simulink model "brakeSystemNeuralNetworkSimulink19b"  (R2021b)
settings: Solver=VariableStepAuto  StartTime=0.0  StopTime=25.0  RelTol=1e-3
settings Model: Creator=hgrady  LastModifiedBy=Nick
settings SolverCC: AlgebraicLoopSolver=TrustRegion

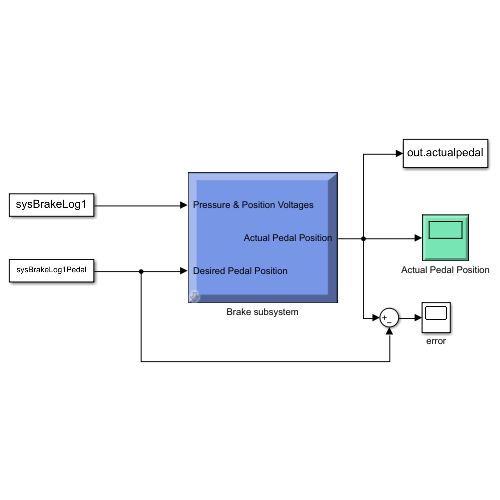
[thumbnail: Simulink's stored preview of the top-level diagram]
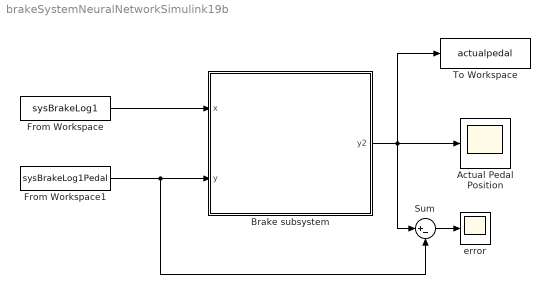
== system brakeSystemNeuralNetworkSimulink19b ==
  Actual Pedal Position : Scope
      mask Display: e = 0.06;c1 = [120 230 180]/255;c2 = ([120 230 180]+0)/(256+128);c3 = ([120 230 180]+128)/(256+128);patch([0 1 1 0],[0 0 1 1],c1);patch([0 1 1 1-e 1-e 0+e],[0 0 1 1-e 0+e 0+e],c2);patch([0 0 1 1-e 0+e 0+e],[0 1 1 1-e 1-e 0+e],c3);plot([0 1 1 0 0],[0 0 1 1 0]);plot([0.15 0.85 0.85 0.15 0.15],[0.5 0.5 0.85 0.85 0.5]);
  Brake subsystem : Subsystem  mask{pi_input_1_delayed_1=[0;0;0;0], pi_input_1_delayed_2=[0;0;0;0], pi_input_1_delayed_3=[0;0;0;0], pi_input_1_delayed_4=[0;0;0;0], pi_input_2_delayed_1=0, pi_input_2_delayed_2=0, pi_input_2_delayed_3=0, pi_input_2_delayed_4=0}
      mask prompts: pi_input_1_delayed_1 "Preprocessed initial input 1 state at timestep 0."; pi_input_1_delayed_2 "Preprocessed initial input 1 state at timestep -1."; pi_input_1_delayed_3 "Preprocessed initial input 1 state at timestep -2."; pi_input_1_delayed_4 "Preprocessed initial input 1 state at timestep -3."; pi_input_2_delayed_1 "Preprocessed initial input 2 state at timestep 0."; pi_input_2_delayed_2 "Preprocessed initial input 2 state at timestep -1."; pi_input_2_delayed_3 "Preprocessed initial input 2 state at timestep -2."; pi_input_2_delayed_4 "Preprocessed initial input 2 state at timestep -3."
      mask help: NARX Neural Network
      mask Display: e = 0.06;c1 = [120 150 230]/255;c2 = ([120 150 230]+0)/383;c3 = ([120 150 230]+128)/383;patch([0 1 1 0],[0 0 1 1],c1);patch([0 1 1 1-e 1-e 0+e],[0 0 1 1-e 0+e 0+e],c2);patch([0 0 1 1-e 0+e 0+e],[0 1 1 1-e 1-e 0+e],c3);plot([0 1 1 0 0],[0 0 1 1 0]);fprintf('');port_label('input',1,' Pressure & Position Voltages');port_label('input',2,' Desired Pedal Position');port_label('output',1,'Actual Pedal Position ');
  From Workspace : FromWorkspace  VariableName=sysBrakeLog1  SampleTime=0.033
  From Workspace1 : FromWorkspace  VariableName=sysBrakeLog1Pedal  SampleTime=0.033
  Sum : Sum  Inputs=|+-
  To Workspace : ToWorkspace  VariableName=actualpedal  SaveFormat=Timeseries  SampleTime=-1
  error : Scope
  wires:
  Brake subsystem/1(y2) -> To Workspace/1, Actual Pedal Position/1, Sum/1
  Sum/1 -> error/1
  From Workspace/1 -> Brake subsystem/1(x)
  From Workspace1/1 -> Brake subsystem/2(y), Sum/2

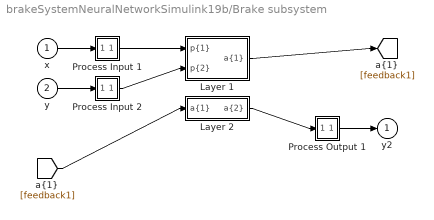
== system brakeSystemNeuralNetworkSimulink19b/Brake subsystem ==
  x : Inport  PortDimensions=4
      mask Display: e = 0.06;c1 = [120 230 180]/255;c2 = ([120 230 180]+0)/(256+128);c3 = ([120 230 180]+128)/(256+128);patch([0 1 1 0],[0 0 1 1],c1);patch([0 1 1 1-e 1-e 0+e],[0 0 1 1-e 0+e 0+e],c2);patch([0 0 1 1-e 0+e 0+e],[0 1 1 1-e 1-e 0+e],c3);plot([0 1 1 0 0],[0 0 1 1 0]);
  y : Inport  Port=2  PortDimensions=1
      mask Display: e = 0.06;c1 = [120 230 180]/255;c2 = ([120 230 180]+0)/(256+128);c3 = ([120 230 180]+128)/(256+128);patch([0 1 1 0],[0 0 1 1],c1);patch([0 1 1 1-e 1-e 0+e],[0 0 1 1-e 0+e 0+e],c2);patch([0 0 1 1-e 0+e 0+e],[0 1 1 1-e 1-e 0+e],c3);plot([0 1 1 0 0],[0 0 1 1 0]);
  Layer 1 : Subsystem
      mask Display: e = 0.06;c1 = [120 150 230]/255;c2 = ([120 150 230]+0)/383;c3 = ([120 150 230]+128)/383;patch([0 1 1 0],[0 0 1 1],c1);patch([0 1 1 1-e 1-e 0+e],[0 0 1 1-e 0+e 0+e],c2);patch([0 0 1 1-e 0+e 0+e],[0 1 1 1-e 1-e 0+e],c3);plot([0 1 1 0 0],[0 0 1 1 0]);
  Layer 2 : Subsystem
      mask Display: e = 0.06;c1 = [120 150 230]/255;c2 = ([120 150 230]+0)/383;c3 = ([120 150 230]+128)/383;patch([0 1 1 0],[0 0 1 1],c1);patch([0 1 1 1-e 1-e 0+e],[0 0 1 1-e 0+e 0+e],c2);patch([0 0 1 1-e 0+e 0+e],[0 1 1 1-e 1-e 0+e],c3);plot([0 1 1 0 0],[0 0 1 1 0]);
  Process Input 1 : Subsystem
      mask Display: e = 0.06;c1 = [120 150 230]/255;c2 = ([120 150 230]+0)/383;c3 = ([120 150 230]+128)/383;patch([0 1 1 0],[0 0 1 1],c1);patch([0 1 1 1-e 1-e 0+e],[0 0 1 1-e 0+e 0+e],c2);patch([0 0 1 1-e 0+e 0+e],[0 1 1 1-e 1-e 0+e],c3);plot([0 1 1 0 0],[0 0 1 1 0]);
  Process Input 2 : Subsystem
      mask Display: e = 0.06;c1 = [120 150 230]/255;c2 = ([120 150 230]+0)/383;c3 = ([120 150 230]+128)/383;patch([0 1 1 0],[0 0 1 1],c1);patch([0 1 1 1-e 1-e 0+e],[0 0 1 1-e 0+e 0+e],c2);patch([0 0 1 1-e 0+e 0+e],[0 1 1 1-e 1-e 0+e],c3);plot([0 1 1 0 0],[0 0 1 1 0]);
  Process Output 1 : Subsystem
      mask Display: e = 0.06;c1 = [120 150 230]/255;c2 = ([120 150 230]+0)/383;c3 = ([120 150 230]+128)/383;patch([0 1 1 0],[0 0 1 1],c1);patch([0 1 1 1-e 1-e 0+e],[0 0 1 1-e 0+e 0+e],c2);patch([0 0 1 1-e 0+e 0+e],[0 1 1 1-e 1-e 0+e],c3);plot([0 1 1 0 0],[0 0 1 1 0]);
  y2 : Outport  InitialOutput=0
      mask Display: e = 0.06;c1 = [120 230 180]/255;c2 = ([120 230 180]+0)/(256+128);c3 = ([120 230 180]+128)/(256+128);patch([0 1 1 0],[0 0 1 1],c1);patch([0 1 1 1-e 1-e 0+e],[0 0 1 1-e 0+e 0+e],c2);patch([0 0 1 1-e 0+e 0+e],[0 1 1 1-e 1-e 0+e],c3);plot([0 1 1 0 0],[0 0 1 1 0]);
  wires:
  x/1 -> Process Input 1/1(x)
  y/1 -> Process Input 2/1(x)
  Process Output 1/1(y) -> y2/1
  Process Input 1/1(p) -> Layer 1/1("p{1}")
  Process Input 2/1(p) -> Layer 1/2("p{2}")
  Layer 1/1("a{1}") -> [feedback1]
  [feedback1] -> Layer 2/1("a{1} ")
  Layer 2/1("a{2}") -> Process Output 1/1(a)

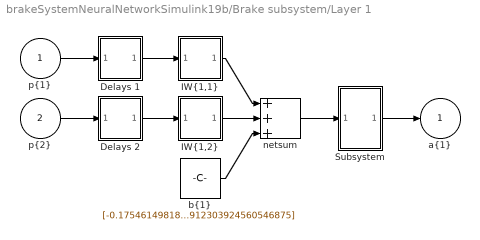
== system brakeSystemNeuralNetworkSimulink19b/Brake subsystem/Layer 1 ==
  "p{1}" : Inport  PortDimensions=4
      mask Display: e = 0.06;c1 = [120 230 180]/255;c2 = ([120 230 180]+0)/(256+128);c3 = ([120 230 180]+128)/(256+128);patch([0 1 1 0],[0 0 1 1],c1);patch([0 1 1 1-e 1-e 0+e],[0 0 1 1-e 0+e 0+e],c2);patch([0 0 1 1-e 0+e 0+e],[0 1 1 1-e 1-e 0+e],c3);plot([0 1 1 0 0],[0 0 1 1 0]);
  "p{2}" : Inport  Port=2  PortDimensions=1
      mask Display: e = 0.06;c1 = [120 230 180]/255;c2 = ([120 230 180]+0)/(256+128);c3 = ([120 230 180]+128)/(256+128);patch([0 1 1 0],[0 0 1 1],c1);patch([0 1 1 1-e 1-e 0+e],[0 0 1 1-e 0+e 0+e],c2);patch([0 0 1 1-e 0+e 0+e],[0 1 1 1-e 1-e 0+e],c3);plot([0 1 1 0 0],[0 0 1 1 0]);
  Delays 1 : Subsystem
      mask Display: e = 0.06;c1 = [120 150 230]/255;c2 = ([120 150 230]+0)/383;c3 = ([120 150 230]+128)/383;patch([0 1 1 0],[0 0 1 1],c1);patch([0 1 1 1-e 1-e 0+e],[0 0 1 1-e 0+e 0+e],c2);patch([0 0 1 1-e 0+e 0+e],[0 1 1 1-e 1-e 0+e],c3);plot([0 1 1 0 0],[0 0 1 1 0]);disp('1-4');
  Delays 2 : Subsystem
      mask Display: e = 0.06;c1 = [120 150 230]/255;c2 = ([120 150 230]+0)/383;c3 = ([120 150 230]+128)/383;patch([0 1 1 0],[0 0 1 1],c1);patch([0 1 1 1-e 1-e 0+e],[0 0 1 1-e 0+e 0+e],c2);patch([0 0 1 1-e 0+e 0+e],[0 1 1 1-e 1-e 0+e],c3);plot([0 1 1 0 0],[0 0 1 1 0]);disp('1-4');
  "IW{1,1}" : Subsystem
      mask Display: e = 0.06;c1 = [120 150 230]/255;c2 = ([120 150 230]+0)/383;c3 = ([120 150 230]+128)/383;patch([0 1 1 0],[0 0 1 1],c1);patch([0 1 1 1-e 1-e 0+e],[0 0 1 1-e 0+e 0+e],c2);patch([0 0 1 1-e 0+e 0+e],[0 1 1 1-e 1-e 0+e],c3);plot([0 1 1 0 0],[0 0 1 1 0]);disp('W');
  "IW{1,2}" : Subsystem
      mask Display: e = 0.06;c1 = [120 150 230]/255;c2 = ([120 150 230]+0)/383;c3 = ([120 150 230]+128)/383;patch([0 1 1 0],[0 0 1 1],c1);patch([0 1 1 1-e 1-e 0+e],[0 0 1 1-e 0+e 0+e],c2);patch([0 0 1 1-e 0+e 0+e],[0 1 1 1-e 1-e 0+e],c3);plot([0 1 1 0 0],[0 0 1 1 0]);disp('W');
  Subsystem : Subsystem
  "b{1}" : Constant  Value=[-0.1754614981831461861805365742839057929813861846923828125;0.1568951812336805973213671450139372609555721282958984375;0.092589380084686812022454205362009815871715545654296875;-0.08827103518596403353146939707585261203348636627197265625;-0.1366947078190251796403487105635576881468296051025390625;-1.6956623977816700499232638321700505912303924560546875]
      mask Display: e = 0.06;c1 = [120 150 230]/255;c2 = ([120 150 230]+0)/383;c3 = ([120 150 230]+128)/383;patch([0 1 1 0],[0 0 1 1],c1);patch([0 1 1 1-e 1-e 0+e],[0 0 1 1-e 0+e 0+e],c2);patch([0 0 1 1-e 0+e 0+e],[0 1 1 1-e 1-e 0+e],c3);plot([0 1 1 0 0],[0 0 1 1 0]);disp('b');
  netsum : Sum  Inputs=3  InputSameDT=on  SaturateOnIntegerOverflow=on  OutDataTypeStr=Inherit: Same as first input
      mask Display: e = 0.06;c1 = [120 150 230]/255;c2 = ([120 150 230]+0)/383;c3 = ([120 150 230]+128)/383;patch([0 1 1 0],[0 0 1 1],c1);patch([0 1 1 1-e 1-e 0+e],[0 0 1 1-e 0+e 0+e],c2);patch([0 0 1 1-e 0+e 0+e],[0 1 1 1-e 1-e 0+e],c3);plot([0 1 1 0 0],[0 0 1 1 0]);disp('+');
  "a{1}" : Outport  InitialOutput=[0;0;0;0;0;0]
      mask Display: e = 0.06;c1 = [120 230 180]/255;c2 = ([120 230 180]+0)/(256+128);c3 = ([120 230 180]+128)/(256+128);patch([0 1 1 0],[0 0 1 1],c1);patch([0 1 1 1-e 1-e 0+e],[0 0 1 1-e 0+e 0+e],c2);patch([0 0 1 1-e 0+e 0+e],[0 1 1 1-e 1-e 0+e],c3);plot([0 1 1 0 0],[0 0 1 1 0]);
  wires:
  "p{1}"/1 -> Delays 1/1("p{1}")
  Delays 1/1("pd{1,1}") -> "IW{1,1}"/1("pd{1,1}")
  "IW{1,1}"/1("iz{1,1}") -> netsum/1
  "p{2}"/1 -> Delays 2/1("p{1}")
  Delays 2/1("pd{1,2}") -> "IW{1,2}"/1("pd{1,2}")
  "IW{1,2}"/1("iz{1,2}") -> netsum/2
  "b{1}"/1 -> netsum/3
  netsum/1 -> Subsystem/1(In1)
  Subsystem/1("a{1}") -> "a{1}"/1

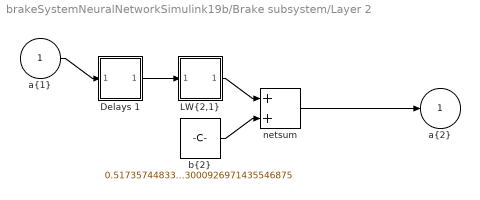
== system brakeSystemNeuralNetworkSimulink19b/Brake subsystem/Layer 2 ==
  "a{1} " : Inport  PortDimensions=6
      mask Display: e = 0.06;c1 = [120 230 180]/255;c2 = ([120 230 180]+0)/(256+128);c3 = ([120 230 180]+128)/(256+128);patch([0 1 1 0],[0 0 1 1],c1);patch([0 1 1 1-e 1-e 0+e],[0 0 1 1-e 0+e 0+e],c2);patch([0 0 1 1-e 0+e 0+e],[0 1 1 1-e 1-e 0+e],c3);plot([0 1 1 0 0],[0 0 1 1 0]);
  Delays 1 : Subsystem
      mask Display: e = 0.06;c1 = [120 150 230]/255;c2 = ([120 150 230]+0)/383;c3 = ([120 150 230]+128)/383;patch([0 1 1 0],[0 0 1 1],c1);patch([0 1 1 1-e 1-e 0+e],[0 0 1 1-e 0+e 0+e],c2);patch([0 0 1 1-e 0+e 0+e],[0 1 1 1-e 1-e 0+e],c3);plot([0 1 1 0 0],[0 0 1 1 0]);disp('0');
  "LW{2,1}" : Subsystem
      mask Display: e = 0.06;c1 = [120 150 230]/255;c2 = ([120 150 230]+0)/383;c3 = ([120 150 230]+128)/383;patch([0 1 1 0],[0 0 1 1],c1);patch([0 1 1 1-e 1-e 0+e],[0 0 1 1-e 0+e 0+e],c2);patch([0 0 1 1-e 0+e 0+e],[0 1 1 1-e 1-e 0+e],c3);plot([0 1 1 0 0],[0 0 1 1 0]);disp('W');
  "b{2}" : Constant  Value=0.51735744833768204653523525848868303000926971435546875
      mask Display: e = 0.06;c1 = [120 150 230]/255;c2 = ([120 150 230]+0)/383;c3 = ([120 150 230]+128)/383;patch([0 1 1 0],[0 0 1 1],c1);patch([0 1 1 1-e 1-e 0+e],[0 0 1 1-e 0+e 0+e],c2);patch([0 0 1 1-e 0+e 0+e],[0 1 1 1-e 1-e 0+e],c3);plot([0 1 1 0 0],[0 0 1 1 0]);disp('b');
  netsum : Sum  Inputs=2  InputSameDT=on  SaturateOnIntegerOverflow=on  OutDataTypeStr=Inherit: Same as first input
      mask Display: e = 0.06;c1 = [120 150 230]/255;c2 = ([120 150 230]+0)/383;c3 = ([120 150 230]+128)/383;patch([0 1 1 0],[0 0 1 1],c1);patch([0 1 1 1-e 1-e 0+e],[0 0 1 1-e 0+e 0+e],c2);patch([0 0 1 1-e 0+e 0+e],[0 1 1 1-e 1-e 0+e],c3);plot([0 1 1 0 0],[0 0 1 1 0]);disp('+');
  "a{2}" : Outport  InitialOutput=0
      mask Display: e = 0.06;c1 = [120 230 180]/255;c2 = ([120 230 180]+0)/(256+128);c3 = ([120 230 180]+128)/(256+128);patch([0 1 1 0],[0 0 1 1],c1);patch([0 1 1 1-e 1-e 0+e],[0 0 1 1-e 0+e 0+e],c2);patch([0 0 1 1-e 0+e 0+e],[0 1 1 1-e 1-e 0+e],c3);plot([0 1 1 0 0],[0 0 1 1 0]);
  wires:
  "a{1} "/1 -> Delays 1/1("p{2}")
  Delays 1/1("pd{2,1}") -> "LW{2,1}"/1("ad{2,1}")
  "LW{2,1}"/1("lz{2,1}") -> netsum/1
  "b{2}"/1 -> netsum/2
  netsum/1 -> "a{2}"/1

== system brakeSystemNeuralNetworkSimulink19b/Brake subsystem/Process Input 1 ==
  x : Inport  PortDimensions=4
      mask Display: e = 0.06;c1 = [120 230 180]/255;c2 = ([120 230 180]+0)/(256+128);c3 = ([120 230 180]+128)/(256+128);patch([0 1 1 0],[0 0 1 1],c1);patch([0 1 1 1-e 1-e 0+e],[0 0 1 1-e 0+e 0+e],c2);patch([0 0 1 1-e 0+e 0+e],[0 1 1 1-e 1-e 0+e],c3);plot([0 1 1 0 0],[0 0 1 1 0]);
  Subsystem : Subsystem
  p : Outport  PortDimensions=4
      mask Display: e = 0.06;c1 = [120 230 180]/255;c2 = ([120 230 180]+0)/(256+128);c3 = ([120 230 180]+128)/(256+128);patch([0 1 1 0],[0 0 1 1],c1);patch([0 1 1 1-e 1-e 0+e],[0 0 1 1-e 0+e 0+e],c2);patch([0 0 1 1-e 0+e 0+e],[0 1 1 1-e 1-e 0+e],c3);plot([0 1 1 0 0],[0 0 1 1 0]);
  wires:
  x/1 -> Subsystem/1(x)
  Subsystem/1(p) -> p/1

== system brakeSystemNeuralNetworkSimulink19b/Brake subsystem/Process Input 2 ==
  x : Inport  PortDimensions=1
      mask Display: e = 0.06;c1 = [120 230 180]/255;c2 = ([120 230 180]+0)/(256+128);c3 = ([120 230 180]+128)/(256+128);patch([0 1 1 0],[0 0 1 1],c1);patch([0 1 1 1-e 1-e 0+e],[0 0 1 1-e 0+e 0+e],c2);patch([0 0 1 1-e 0+e 0+e],[0 1 1 1-e 1-e 0+e],c3);plot([0 1 1 0 0],[0 0 1 1 0]);
  Subsystem : Subsystem
  p : Outport  PortDimensions=1
      mask Display: e = 0.06;c1 = [120 230 180]/255;c2 = ([120 230 180]+0)/(256+128);c3 = ([120 230 180]+128)/(256+128);patch([0 1 1 0],[0 0 1 1],c1);patch([0 1 1 1-e 1-e 0+e],[0 0 1 1-e 0+e 0+e],c2);patch([0 0 1 1-e 0+e 0+e],[0 1 1 1-e 1-e 0+e],c3);plot([0 1 1 0 0],[0 0 1 1 0]);
  wires:
  Subsystem/1(p) -> p/1
  x/1 -> Subsystem/1(x)

== system brakeSystemNeuralNetworkSimulink19b/Brake subsystem/Process Output 1 ==
  a : Inport  PortDimensions=1
      mask Display: e = 0.06;c1 = [120 230 180]/255;c2 = ([120 230 180]+0)/(256+128);c3 = ([120 230 180]+128)/(256+128);patch([0 1 1 0],[0 0 1 1],c1);patch([0 1 1 1-e 1-e 0+e],[0 0 1 1-e 0+e 0+e],c2);patch([0 0 1 1-e 0+e 0+e],[0 1 1 1-e 1-e 0+e],c3);plot([0 1 1 0 0],[0 0 1 1 0]);
  Subsystem : Subsystem
  y : Outport  PortDimensions=1
      mask Display: e = 0.06;c1 = [120 230 180]/255;c2 = ([120 230 180]+0)/(256+128);c3 = ([120 230 180]+128)/(256+128);patch([0 1 1 0],[0 0 1 1],c1);patch([0 1 1 1-e 1-e 0+e],[0 0 1 1-e 0+e 0+e],c2);patch([0 0 1 1-e 0+e 0+e],[0 1 1 1-e 1-e 0+e],c3);plot([0 1 1 0 0],[0 0 1 1 0]);
  wires:
  a/1 -> Subsystem/1(a)
  Subsystem/1(y) -> y/1

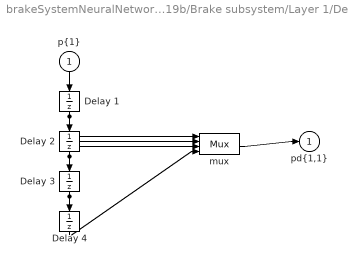
== system brakeSystemNeuralNetworkSimulink19b/Brake subsystem/Layer 1/Delays 1 ==
  "p{1}" : Inport  PortDimensions=4
      mask Display: e = 0.06;c1 = [120 230 180]/255;c2 = ([120 230 180]+0)/(256+128);c3 = ([120 230 180]+128)/(256+128);patch([0 1 1 0],[0 0 1 1],c1);patch([0 1 1 1-e 1-e 0+e],[0 0 1 1-e 0+e 0+e],c2);patch([0 0 1 1-e 0+e 0+e],[0 1 1 1-e 1-e 0+e],c3);plot([0 1 1 0 0],[0 0 1 1 0]);
  Delay 1 : UnitDelay  InitialCondition=pi_input_1_delayed_1  SampleTime=-1
      mask Display: e = 0.06;c1 = [120 150 230]/255;c2 = ([120 150 230]+0)/383;c3 = ([120 150 230]+128)/383;patch([0 1 1 0],[0 0 1 1],c1);patch([0 1 1 1-e 1-e 0+e],[0 0 1 1-e 0+e 0+e],c2);patch([0 0 1 1-e 0+e 0+e],[0 1 1 1-e 1-e 0+e],c3);plot([0 1 1 0 0],[0 0 1 1 0]);disp('D')
  Delay 2 : UnitDelay  InitialCondition=pi_input_1_delayed_2  SampleTime=-1
      mask Display: e = 0.06;c1 = [120 150 230]/255;c2 = ([120 150 230]+0)/383;c3 = ([120 150 230]+128)/383;patch([0 1 1 0],[0 0 1 1],c1);patch([0 1 1 1-e 1-e 0+e],[0 0 1 1-e 0+e 0+e],c2);patch([0 0 1 1-e 0+e 0+e],[0 1 1 1-e 1-e 0+e],c3);plot([0 1 1 0 0],[0 0 1 1 0]);disp('D')
  Delay 3 : UnitDelay  InitialCondition=pi_input_1_delayed_3  SampleTime=-1
      mask Display: e = 0.06;c1 = [120 150 230]/255;c2 = ([120 150 230]+0)/383;c3 = ([120 150 230]+128)/383;patch([0 1 1 0],[0 0 1 1],c1);patch([0 1 1 1-e 1-e 0+e],[0 0 1 1-e 0+e 0+e],c2);patch([0 0 1 1-e 0+e 0+e],[0 1 1 1-e 1-e 0+e],c3);plot([0 1 1 0 0],[0 0 1 1 0]);disp('D')
  Delay 4 : UnitDelay  InitialCondition=pi_input_1_delayed_4  SampleTime=-1
      mask Display: e = 0.06;c1 = [120 150 230]/255;c2 = ([120 150 230]+0)/383;c3 = ([120 150 230]+128)/383;patch([0 1 1 0],[0 0 1 1],c1);patch([0 1 1 1-e 1-e 0+e],[0 0 1 1-e 0+e 0+e],c2);patch([0 0 1 1-e 0+e 0+e],[0 1 1 1-e 1-e 0+e],c3);plot([0 1 1 0 0],[0 0 1 1 0]);disp('D')
  mux : Mux
      mask Display: e = 0.06;c1 = [120 150 230]/255;c2 = ([120 150 230]+0)/383;c3 = ([120 150 230]+128)/383;patch([0 1 1 0],[0 0 1 1],c1);patch([0 1 1 1-e 1-e 0+e],[0 0 1 1-e 0+e 0+e],c2);patch([0 0 1 1-e 0+e 0+e],[0 1 1 1-e 1-e 0+e],c3);plot([0 1 1 0 0],[0 0 1 1 0]);disp('Mux')
  "pd{1,1}" : Outport
      mask Display: e = 0.06;c1 = [120 230 180]/255;c2 = ([120 230 180]+0)/(256+128);c3 = ([120 230 180]+128)/(256+128);patch([0 1 1 0],[0 0 1 1],c1);patch([0 1 1 1-e 1-e 0+e],[0 0 1 1-e 0+e 0+e],c2);patch([0 0 1 1-e 0+e 0+e],[0 1 1 1-e 1-e 0+e],c3);plot([0 1 1 0 0],[0 0 1 1 0]);
  wires:
  "p{1}"/1 -> Delay 1/1
  Delay 1/1 -> Delay 2/1, mux/1
  Delay 2/1 -> Delay 3/1, mux/2
  Delay 3/1 -> Delay 4/1, mux/3
  Delay 4/1 -> mux/4
  mux/1 -> "pd{1,1}"/1

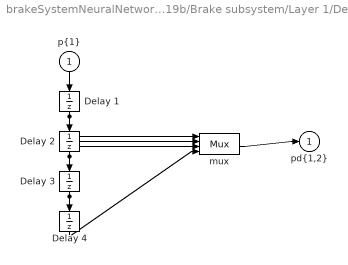
== system brakeSystemNeuralNetworkSimulink19b/Brake subsystem/Layer 1/Delays 2 ==
  "p{1}" : Inport  PortDimensions=1
      mask Display: e = 0.06;c1 = [120 230 180]/255;c2 = ([120 230 180]+0)/(256+128);c3 = ([120 230 180]+128)/(256+128);patch([0 1 1 0],[0 0 1 1],c1);patch([0 1 1 1-e 1-e 0+e],[0 0 1 1-e 0+e 0+e],c2);patch([0 0 1 1-e 0+e 0+e],[0 1 1 1-e 1-e 0+e],c3);plot([0 1 1 0 0],[0 0 1 1 0]);
  Delay 1 : UnitDelay  InitialCondition=pi_input_2_delayed_1  SampleTime=-1
      mask Display: e = 0.06;c1 = [120 150 230]/255;c2 = ([120 150 230]+0)/383;c3 = ([120 150 230]+128)/383;patch([0 1 1 0],[0 0 1 1],c1);patch([0 1 1 1-e 1-e 0+e],[0 0 1 1-e 0+e 0+e],c2);patch([0 0 1 1-e 0+e 0+e],[0 1 1 1-e 1-e 0+e],c3);plot([0 1 1 0 0],[0 0 1 1 0]);disp('D')
  Delay 2 : UnitDelay  InitialCondition=pi_input_2_delayed_2  SampleTime=-1
      mask Display: e = 0.06;c1 = [120 150 230]/255;c2 = ([120 150 230]+0)/383;c3 = ([120 150 230]+128)/383;patch([0 1 1 0],[0 0 1 1],c1);patch([0 1 1 1-e 1-e 0+e],[0 0 1 1-e 0+e 0+e],c2);patch([0 0 1 1-e 0+e 0+e],[0 1 1 1-e 1-e 0+e],c3);plot([0 1 1 0 0],[0 0 1 1 0]);disp('D')
  Delay 3 : UnitDelay  InitialCondition=pi_input_2_delayed_3  SampleTime=-1
      mask Display: e = 0.06;c1 = [120 150 230]/255;c2 = ([120 150 230]+0)/383;c3 = ([120 150 230]+128)/383;patch([0 1 1 0],[0 0 1 1],c1);patch([0 1 1 1-e 1-e 0+e],[0 0 1 1-e 0+e 0+e],c2);patch([0 0 1 1-e 0+e 0+e],[0 1 1 1-e 1-e 0+e],c3);plot([0 1 1 0 0],[0 0 1 1 0]);disp('D')
  Delay 4 : UnitDelay  InitialCondition=pi_input_2_delayed_4  SampleTime=-1
      mask Display: e = 0.06;c1 = [120 150 230]/255;c2 = ([120 150 230]+0)/383;c3 = ([120 150 230]+128)/383;patch([0 1 1 0],[0 0 1 1],c1);patch([0 1 1 1-e 1-e 0+e],[0 0 1 1-e 0+e 0+e],c2);patch([0 0 1 1-e 0+e 0+e],[0 1 1 1-e 1-e 0+e],c3);plot([0 1 1 0 0],[0 0 1 1 0]);disp('D')
  mux : Mux
      mask Display: e = 0.06;c1 = [120 150 230]/255;c2 = ([120 150 230]+0)/383;c3 = ([120 150 230]+128)/383;patch([0 1 1 0],[0 0 1 1],c1);patch([0 1 1 1-e 1-e 0+e],[0 0 1 1-e 0+e 0+e],c2);patch([0 0 1 1-e 0+e 0+e],[0 1 1 1-e 1-e 0+e],c3);plot([0 1 1 0 0],[0 0 1 1 0]);disp('Mux')
  "pd{1,2}" : Outport
      mask Display: e = 0.06;c1 = [120 230 180]/255;c2 = ([120 230 180]+0)/(256+128);c3 = ([120 230 180]+128)/(256+128);patch([0 1 1 0],[0 0 1 1],c1);patch([0 1 1 1-e 1-e 0+e],[0 0 1 1-e 0+e 0+e],c2);patch([0 0 1 1-e 0+e 0+e],[0 1 1 1-e 1-e 0+e],c3);plot([0 1 1 0 0],[0 0 1 1 0]);
  wires:
  "p{1}"/1 -> Delay 1/1
  Delay 1/1 -> Delay 2/1, mux/1
  Delay 2/1 -> Delay 3/1, mux/2
  Delay 3/1 -> Delay 4/1, mux/3
  Delay 4/1 -> mux/4
  mux/1 -> "pd{1,2}"/1

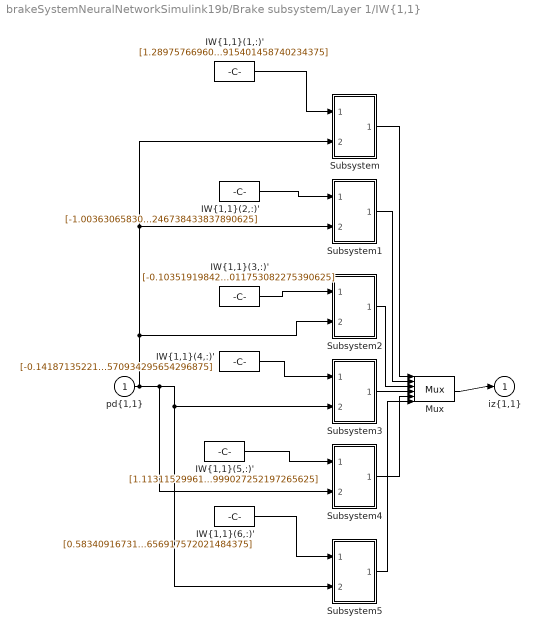
== system brakeSystemNeuralNetworkSimulink19b/Brake subsystem/Layer 1/IW{1,1} ==
  "pd{1,1}" : Inport  PortDimensions=16
      mask Display: e = 0.06;c1 = [120 230 180]/255;c2 = ([120 230 180]+0)/(256+128);c3 = ([120 230 180]+128)/(256+128);patch([0 1 1 0],[0 0 1 1],c1);patch([0 1 1 1-e 1-e 0+e],[0 0 1 1-e 0+e 0+e],c2);patch([0 0 1 1-e 0+e 0+e],[0 1 1 1-e 1-e 0+e],c3);plot([0 1 1 0 0],[0 0 1 1 0]);
  "IW{1,1}(1,:)'" : Constant  Value=[1.2897576696065213841535523897618986666202545166015625;-1.9225315294228157991796024361974559724330902099609375;-0.00402625356027518956081312495598467648960649967193603515625;-0.0988800330330607823992039584481972269713878631591796875;-0.27745355869966548123528582436847500503063201904296875;-0.12242203843162434429014950865166611038148403167724609375;0.045299790642422767261709992681062431074678897857666015625;0.2322400561246042161034353057402768172323703765869140625;0.540012487374641469983771457918919622898101806640625;-0.317979220729676381740347324011963792145252227783203125;-0.071153555664597967211904006035183556377887725830078125;0.6664762409444053847806799240061081945896148681640625;-0.10006387485759764277570837975872564129531383514404296875;1.1585855314879764943469808713416568934917449951171875;-1.066665946007540721751638557179830968379974365234375;0.2126378942000091976094466872382326982915401458740234375]
      mask Display: e = 0.06;c1 = [120 150 230]/255;c2 = ([120 150 230]+0)/383;c3 = ([120 150 230]+128)/383;patch([0 1 1 0],[0 0 1 1],c1);patch([0 1 1 1-e 1-e 0+e],[0 0 1 1-e 0+e 0+e],c2);patch([0 0 1 1-e 0+e 0+e],[0 1 1 1-e 1-e 0+e],c3);plot([0 1 1 0 0],[0 0 1 1 0]);disp('Weights');
  "IW{1,1}(2,:)'" : Constant  Value=[-1.003630658309852652365634639863856136798858642578125;0.338523526913924677206324531653081066906452178955078125;0.9422901927147353529079509826260618865489959716796875;-1.1446515869217623873055345029570162296295166015625;-0.343800873428868170034178319838247261941432952880859375;0.73667385246239625029573971914942376315593719482421875;1.2733273896138239678066383930854499340057373046875;-0.870093591850880532234668862656690180301666259765625;-0.2120035384527268751408968228133744560182094573974609375;0.43020063762066829138319690173375420272350311279296875;0.358071043315450976418645723242661915719509124755859375;-0.2214202339524725948738392844461486674845218658447265625;1.0166826058251110520558313510264270007610321044921875;-0.98900030881367839707962730244616977870464324951171875;-1.426959764997298929500857411767356097698211669921875;1.1970974616296192749587135040201246738433837890625]
      mask Display: e = 0.06;c1 = [120 150 230]/255;c2 = ([120 150 230]+0)/383;c3 = ([120 150 230]+128)/383;patch([0 1 1 0],[0 0 1 1],c1);patch([0 1 1 1-e 1-e 0+e],[0 0 1 1-e 0+e 0+e],c2);patch([0 0 1 1-e 0+e 0+e],[0 1 1 1-e 1-e 0+e],c3);plot([0 1 1 0 0],[0 0 1 1 0]);disp('Weights');
  "IW{1,1}(3,:)'" : Constant  Value=[-0.10351919842323031861752724580583162605762481689453125;-0.291936673311472161262969393646926619112491607666015625;0.342352126239464926715783121835556812584400177001953125;-0.3225497432442183676215563536970876157283782958984375;0.073595415211766823659900182974524796009063720703125;0.330315580923162432913642305720713920891284942626953125;0.2319635581233006338397473200529930181801319122314453125;-0.1457676472005481060900677903191535733640193939208984375;-0.12028815781712472177122918992608902044594287872314453125;0.451619436440927002340828266824246384203433990478515625;-0.0184090182338133602490959361830391571857035160064697265625;-0.13889567432849669881278487082454375922679901123046875;0.369567014014314965120178158031194470822811126708984375;0.2577282676341869915859206230379641056060791015625;-0.5734592179285709079294974799267947673797607421875;0.51829775585077531019351226859726011753082275390625]
      mask Display: e = 0.06;c1 = [120 150 230]/255;c2 = ([120 150 230]+0)/383;c3 = ([120 150 230]+128)/383;patch([0 1 1 0],[0 0 1 1],c1);patch([0 1 1 1-e 1-e 0+e],[0 0 1 1-e 0+e 0+e],c2);patch([0 0 1 1-e 0+e 0+e],[0 1 1 1-e 1-e 0+e],c3);plot([0 1 1 0 0],[0 0 1 1 0]);disp('Weights');
  "IW{1,1}(4,:)'" : Constant  Value=[-0.141871352218838564507308319662115536630153656005859375;-0.85302991194646693440262197327683679759502410888671875;0.08385365033729719197452823209459893405437469482421875;-0.36003567776693190527481647222884930670261383056640625;0.0860344640610527233715032480176887474954128265380859375;0.67341138358948071651610689514200203120708465576171875;0.0620439414085031948342674468221957795321941375732421875;0.183522153508646257424885561704286374151706695556640625;-0.6642097780102791393375127881881780922412872314453125;0.56547880886903933994602766688331030309200286865234375;-0.2998612243139604505159923064638860523700714111328125;-0.31440704378714101618896847867290489375591278076171875;-0.08020721694382017263880157997846254147589206695556640625;0.73182407544959138245843632830656133592128753662109375;-0.6999964065276607083632143258000724017620086669921875;1.0924587938600101022501576153445057570934295654296875]
      mask Display: e = 0.06;c1 = [120 150 230]/255;c2 = ([120 150 230]+0)/383;c3 = ([120 150 230]+128)/383;patch([0 1 1 0],[0 0 1 1],c1);patch([0 1 1 1-e 1-e 0+e],[0 0 1 1-e 0+e 0+e],c2);patch([0 0 1 1-e 0+e 0+e],[0 1 1 1-e 1-e 0+e],c3);plot([0 1 1 0 0],[0 0 1 1 0]);disp('Weights');
  "IW{1,1}(5,:)'" : Constant  Value=[1.113115299612319919475567076005972921848297119140625;-0.9035501960938343568585651155444793403148651123046875;-0.13889190081698143952593227368197403848171234130859375;0.433101759647144479714597764541395008563995361328125;0.16612749920642588818964213714934885501861572265625;-0.463801286601643270035566501974244602024555206298828125;-0.488628247025082840249154969569644890725612640380859375;0.32850827051545328227888376204646192491054534912109375;0.6087789402608507760561451505054719746112823486328125;-0.0900418699435361069571825964885647408664226531982421875;-0.10450239558573588827261602318685618229210376739501953125;0.420199543608407444228447502609924413263797760009765625;-0.06908799165002156572601421657964237965643405914306640625;1.016205292184789499287944636307656764984130859375;0.047350876092135167627628078435009228996932506561279296875;-0.5856513790872475144766440280363894999027252197265625]
      mask Display: e = 0.06;c1 = [120 150 230]/255;c2 = ([120 150 230]+0)/383;c3 = ([120 150 230]+128)/383;patch([0 1 1 0],[0 0 1 1],c1);patch([0 1 1 1-e 1-e 0+e],[0 0 1 1-e 0+e 0+e],c2);patch([0 0 1 1-e 0+e 0+e],[0 1 1 1-e 1-e 0+e],c3);plot([0 1 1 0 0],[0 0 1 1 0]);disp('Weights');
  "IW{1,1}(6,:)'" : Constant  Value=[0.58340916731774739023563824957818724215030670166015625;-1.471002313660239479986557853408157825469970703125;-0.048550598771022031308053357179232989437878131866455078125;-0.82705537176623244999262851706589572131633758544921875;0.2131262359346118018255111792313982732594013214111328125;1.0493438587754908564164679773966781795024871826171875;-0.7026456738917501443353330614627338945865631103515625;1.5306766640341591401153209517360664904117584228515625;-0.4287376990170408408431512725655920803546905517578125;1.325926437278113656503819584031589329242706298828125;-1.2972397716879806583989420687430538237094879150390625;0.413967425034627634072847968127462081611156463623046875;1.1652572398799707631411592956283129751682281494140625;1.4338241335849029045590441455715335905551910400390625;-1.8739474430102347479731861312757246196269989013671875;1.9561367062098911073775298063992522656917572021484375]
      mask Display: e = 0.06;c1 = [120 150 230]/255;c2 = ([120 150 230]+0)/383;c3 = ([120 150 230]+128)/383;patch([0 1 1 0],[0 0 1 1],c1);patch([0 1 1 1-e 1-e 0+e],[0 0 1 1-e 0+e 0+e],c2);patch([0 0 1 1-e 0+e 0+e],[0 1 1 1-e 1-e 0+e],c3);plot([0 1 1 0 0],[0 0 1 1 0]);disp('Weights');
  Mux : Mux  Inputs=6
      mask Display: e = 0.06;c1 = [120 150 230]/255;c2 = ([120 150 230]+0)/383;c3 = ([120 150 230]+128)/383;patch([0 1 1 0],[0 0 1 1],c1);patch([0 1 1 1-e 1-e 0+e],[0 0 1 1-e 0+e 0+e],c2);patch([0 0 1 1-e 0+e 0+e],[0 1 1 1-e 1-e 0+e],c3);plot([0 1 1 0 0],[0 0 1 1 0]);disp('Mux');
  Subsystem : Subsystem
  Subsystem1 : Subsystem
  Subsystem2 : Subsystem
  Subsystem3 : Subsystem
  Subsystem4 : Subsystem
  Subsystem5 : Subsystem
  "iz{1,1}" : Outport
      mask Display: e = 0.06;c1 = [120 230 180]/255;c2 = ([120 230 180]+0)/(256+128);c3 = ([120 230 180]+128)/(256+128);patch([0 1 1 0],[0 0 1 1],c1);patch([0 1 1 1-e 1-e 0+e],[0 0 1 1-e 0+e 0+e],c2);patch([0 0 1 1-e 0+e 0+e],[0 1 1 1-e 1-e 0+e],c3);plot([0 1 1 0 0],[0 0 1 1 0]);
  wires:
  "pd{1,1}"/1 -> Subsystem1/2("pd{1,1}"), Subsystem/2("pd{1,1}"), Subsystem2/2("pd{1,1}"), Subsystem4/2("pd{1,1}"), Subsystem5/2("pd{1,1}"), Subsystem3/2("pd{1,1}")
  Mux/1 -> "iz{1,1}"/1
  "IW{1,1}(1,:)'"/1 -> Subsystem/1(In1)
  Subsystem/1(Out1) -> Mux/1
  "IW{1,1}(2,:)'"/1 -> Subsystem1/1(In1)
  Subsystem1/1(Out1) -> Mux/2
  "IW{1,1}(3,:)'"/1 -> Subsystem2/1(In1)
  Subsystem2/1(Out1) -> Mux/3
  "IW{1,1}(4,:)'"/1 -> Subsystem3/1(In1)
  Subsystem3/1(Out1) -> Mux/4
  "IW{1,1}(5,:)'"/1 -> Subsystem4/1(In1)
  Subsystem4/1(Out1) -> Mux/5
  "IW{1,1}(6,:)'"/1 -> Subsystem5/1(In1)
  Subsystem5/1(Out1) -> Mux/6

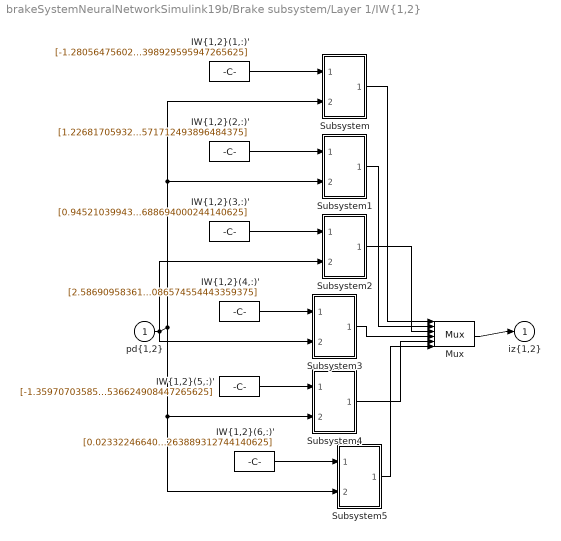
== system brakeSystemNeuralNetworkSimulink19b/Brake subsystem/Layer 1/IW{1,2} ==
  "pd{1,2}" : Inport  PortDimensions=4
      mask Display: e = 0.06;c1 = [120 230 180]/255;c2 = ([120 230 180]+0)/(256+128);c3 = ([120 230 180]+128)/(256+128);patch([0 1 1 0],[0 0 1 1],c1);patch([0 1 1 1-e 1-e 0+e],[0 0 1 1-e 0+e 0+e],c2);patch([0 0 1 1-e 0+e 0+e],[0 1 1 1-e 1-e 0+e],c3);plot([0 1 1 0 0],[0 0 1 1 0]);
  "IW{1,2}(1,:)'" : Constant  Value=[-1.2805647560202559898101526414393447339534759521484375;-0.9036662676938984617436290136538445949554443359375;1.3116465208219298954617215713369660079479217529296875;-1.4052859676147113621169637553975917398929595947265625]
      mask Display: e = 0.06;c1 = [120 150 230]/255;c2 = ([120 150 230]+0)/383;c3 = ([120 150 230]+128)/383;patch([0 1 1 0],[0 0 1 1],c1);patch([0 1 1 1-e 1-e 0+e],[0 0 1 1-e 0+e 0+e],c2);patch([0 0 1 1-e 0+e 0+e],[0 1 1 1-e 1-e 0+e],c3);plot([0 1 1 0 0],[0 0 1 1 0]);disp('Weights');
  "IW{1,2}(2,:)'" : Constant  Value=[1.2268170593222491593365930384607054293155670166015625;-0.52351574333652439730002470241743139922618865966796875;2.65267753497795322203955947770737111568450927734375;-2.57004332534800905563088235794566571712493896484375]
      mask Display: e = 0.06;c1 = [120 150 230]/255;c2 = ([120 150 230]+0)/383;c3 = ([120 150 230]+128)/383;patch([0 1 1 0],[0 0 1 1],c1);patch([0 1 1 1-e 1-e 0+e],[0 0 1 1-e 0+e 0+e],c2);patch([0 0 1 1-e 0+e 0+e],[0 1 1 1-e 1-e 0+e],c3);plot([0 1 1 0 0],[0 0 1 1 0]);disp('Weights');
  "IW{1,2}(3,:)'" : Constant  Value=[0.9452103994355611771283065536408685147762298583984375;-0.36696566846617206802960708955652080476284027099609375;1.036830608888795079991496095317415893077850341796875;-1.2461929722797382424914758303202688694000244140625]
      mask Display: e = 0.06;c1 = [120 150 230]/255;c2 = ([120 150 230]+0)/383;c3 = ([120 150 230]+128)/383;patch([0 1 1 0],[0 0 1 1],c1);patch([0 1 1 1-e 1-e 0+e],[0 0 1 1-e 0+e 0+e],c2);patch([0 0 1 1-e 0+e 0+e],[0 1 1 1-e 1-e 0+e],c3);plot([0 1 1 0 0],[0 0 1 1 0]);disp('Weights');
  "IW{1,2}(4,:)'" : Constant  Value=[2.58690958361750578120563659467734396457672119140625;0.05243374299671281490997643004448036663234233856201171875;1.5982070701513848565156195036252029240131378173828125;-2.25582669569761318228984237066470086574554443359375]
      mask Display: e = 0.06;c1 = [120 150 230]/255;c2 = ([120 150 230]+0)/383;c3 = ([120 150 230]+128)/383;patch([0 1 1 0],[0 0 1 1],c1);patch([0 1 1 1-e 1-e 0+e],[0 0 1 1-e 0+e 0+e],c2);patch([0 0 1 1-e 0+e 0+e],[0 1 1 1-e 1-e 0+e],c3);plot([0 1 1 0 0],[0 0 1 1 0]);disp('Weights');
  "IW{1,2}(5,:)'" : Constant  Value=[-1.359707035850025391710005351342260837554931640625;-0.61556878643991763677689732503495179116725921630859375;-0.577309152811082970657707846839912235736846923828125;0.6164466862102335742434888743446208536624908447265625]
      mask Display: e = 0.06;c1 = [120 150 230]/255;c2 = ([120 150 230]+0)/383;c3 = ([120 150 230]+128)/383;patch([0 1 1 0],[0 0 1 1],c1);patch([0 1 1 1-e 1-e 0+e],[0 0 1 1-e 0+e 0+e],c2);patch([0 0 1 1-e 0+e 0+e],[0 1 1 1-e 1-e 0+e],c3);plot([0 1 1 0 0],[0 0 1 1 0]);disp('Weights');
  "IW{1,2}(6,:)'" : Constant  Value=[0.02332246640720410379987725946193677373230457305908203125;-1.4878855971233146959775694995187222957611083984375;0.71583171766138053992989398466306738555431365966796875;-0.1776705066679158395714921425678767263889312744140625]
      mask Display: e = 0.06;c1 = [120 150 230]/255;c2 = ([120 150 230]+0)/383;c3 = ([120 150 230]+128)/383;patch([0 1 1 0],[0 0 1 1],c1);patch([0 1 1 1-e 1-e 0+e],[0 0 1 1-e 0+e 0+e],c2);patch([0 0 1 1-e 0+e 0+e],[0 1 1 1-e 1-e 0+e],c3);plot([0 1 1 0 0],[0 0 1 1 0]);disp('Weights');
  Mux : Mux  Inputs=6
      mask Display: e = 0.06;c1 = [120 150 230]/255;c2 = ([120 150 230]+0)/383;c3 = ([120 150 230]+128)/383;patch([0 1 1 0],[0 0 1 1],c1);patch([0 1 1 1-e 1-e 0+e],[0 0 1 1-e 0+e 0+e],c2);patch([0 0 1 1-e 0+e 0+e],[0 1 1 1-e 1-e 0+e],c3);plot([0 1 1 0 0],[0 0 1 1 0]);disp('Mux');
  Subsystem : Subsystem
  Subsystem1 : Subsystem
  Subsystem2 : Subsystem
  Subsystem3 : Subsystem
  Subsystem4 : Subsystem
  Subsystem5 : Subsystem
  "iz{1,2}" : Outport
      mask Display: e = 0.06;c1 = [120 230 180]/255;c2 = ([120 230 180]+0)/(256+128);c3 = ([120 230 180]+128)/(256+128);patch([0 1 1 0],[0 0 1 1],c1);patch([0 1 1 1-e 1-e 0+e],[0 0 1 1-e 0+e 0+e],c2);patch([0 0 1 1-e 0+e 0+e],[0 1 1 1-e 1-e 0+e],c3);plot([0 1 1 0 0],[0 0 1 1 0]);
  wires:
  "pd{1,2}"/1 -> Subsystem3/2("pd{1,2}"), Subsystem5/2("pd{1,2}"), Subsystem4/2("pd{1,2}"), Subsystem1/2("pd{1,2}"), Subsystem/2("pd{1,2}"), Subsystem2/2("pd{1,2}")
  Mux/1 -> "iz{1,2}"/1
  "IW{1,2}(1,:)'"/1 -> Subsystem/1(In1)
  Subsystem/1(Out1) -> Mux/1
  "IW{1,2}(2,:)'"/1 -> Subsystem1/1(In1)
  Subsystem1/1(Out1) -> Mux/2
  "IW{1,2}(3,:)'"/1 -> Subsystem2/1(In1)
  Subsystem2/1(Out1) -> Mux/3
  "IW{1,2}(4,:)'"/1 -> Subsystem3/1(In1)
  Subsystem3/1(Out1) -> Mux/4
  "IW{1,2}(5,:)'"/1 -> Subsystem4/1(In1)
  Subsystem4/1(Out1) -> Mux/5
  "IW{1,2}(6,:)'"/1 -> Subsystem5/1(In1)
  Subsystem5/1(Out1) -> Mux/6

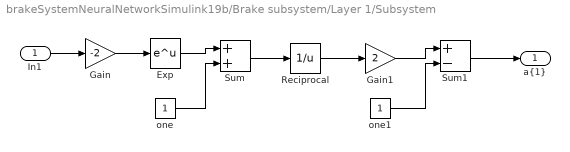
== system brakeSystemNeuralNetworkSimulink19b/Brake subsystem/Layer 1/Subsystem ==
  In1 : Inport
  Exp : Math  SignedPower=on  SaturateOnIntegerOverflow=on
  Gain : Gain  Gain=-2  SaturateOnIntegerOverflow=on  OutDataTypeStr=Inherit: Same as input  ParamDataTypeStr=Inherit: Same as input
  Gain1 : Gain  Gain=2  SaturateOnIntegerOverflow=on  OutDataTypeStr=Inherit: Same as input  ParamDataTypeStr=Inherit: Same as input
  Reciprocal : Math  Operator=reciprocal  SignedPower=on  SaturateOnIntegerOverflow=on
  Sum : Sum  InputSameDT=on  SaturateOnIntegerOverflow=on  OutDataTypeStr=Inherit: Same as first input
  Sum1 : Sum  Inputs=+-  InputSameDT=on  SaturateOnIntegerOverflow=on  OutDataTypeStr=Inherit: Same as first input
  one : Constant
  one1 : Constant
  "a{1}" : Outport
  wires:
  Gain/1 -> Exp/1
  Exp/1 -> Sum/1
  Sum1/1 -> "a{1}"/1
  Reciprocal/1 -> Gain1/1
  Sum/1 -> Reciprocal/1
  one1/1 -> Sum1/2
  Gain1/1 -> Sum1/1
  one/1 -> Sum/2
  In1/1 -> Gain/1

== system brakeSystemNeuralNetworkSimulink19b/Brake subsystem/Layer 2/Delays 1 ==
  "p{2}" : Inport  PortDimensions=6
      mask Display: e = 0.06;c1 = [120 230 180]/255;c2 = ([120 230 180]+0)/(256+128);c3 = ([120 230 180]+128)/(256+128);patch([0 1 1 0],[0 0 1 1],c1);patch([0 1 1 1-e 1-e 0+e],[0 0 1 1-e 0+e 0+e],c2);patch([0 0 1 1-e 0+e 0+e],[0 1 1 1-e 1-e 0+e],c3);plot([0 1 1 0 0],[0 0 1 1 0]);
  mux : Mux  Inputs=1
      mask Display: e = 0.06;c1 = [120 150 230]/255;c2 = ([120 150 230]+0)/383;c3 = ([120 150 230]+128)/383;patch([0 1 1 0],[0 0 1 1],c1);patch([0 1 1 1-e 1-e 0+e],[0 0 1 1-e 0+e 0+e],c2);patch([0 0 1 1-e 0+e 0+e],[0 1 1 1-e 1-e 0+e],c3);plot([0 1 1 0 0],[0 0 1 1 0]);disp('Mux')
  "pd{2,1}" : Outport
      mask Display: e = 0.06;c1 = [120 230 180]/255;c2 = ([120 230 180]+0)/(256+128);c3 = ([120 230 180]+128)/(256+128);patch([0 1 1 0],[0 0 1 1],c1);patch([0 1 1 1-e 1-e 0+e],[0 0 1 1-e 0+e 0+e],c2);patch([0 0 1 1-e 0+e 0+e],[0 1 1 1-e 1-e 0+e],c3);plot([0 1 1 0 0],[0 0 1 1 0]);
  wires:
  "p{2}"/1 -> mux/1
  mux/1 -> "pd{2,1}"/1

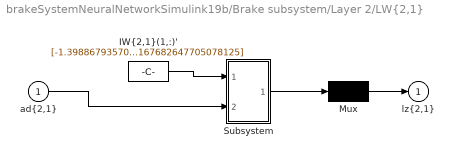
== system brakeSystemNeuralNetworkSimulink19b/Brake subsystem/Layer 2/LW{2,1} ==
  "ad{2,1}" : Inport  PortDimensions=6
      mask Display: e = 0.06;c1 = [120 230 180]/255;c2 = ([120 230 180]+0)/(256+128);c3 = ([120 230 180]+128)/(256+128);patch([0 1 1 0],[0 0 1 1],c1);patch([0 1 1 1-e 1-e 0+e],[0 0 1 1-e 0+e 0+e],c2);patch([0 0 1 1-e 0+e 0+e],[0 1 1 1-e 1-e 0+e],c3);plot([0 1 1 0 0],[0 0 1 1 0]);
  "IW{2,1}(1,:)'" : Constant  Value=[-1.398867935704070308844393366598524153232574462890625;2.143929645762529645480753970332443714141845703125;-5.13675642106006336007339996285736560821533203125;2.1922784606724832201507524587213993072509765625;3.37769993167163473657410577288828790187835693359375;-0.06339503179608670102584966343783889897167682647705078125]
      mask Display: e = 0.06;c1 = [120 150 230]/255;c2 = ([120 150 230]+0)/383;c3 = ([120 150 230]+128)/383;patch([0 1 1 0],[0 0 1 1],c1);patch([0 1 1 1-e 1-e 0+e],[0 0 1 1-e 0+e 0+e],c2);patch([0 0 1 1-e 0+e 0+e],[0 1 1 1-e 1-e 0+e],c3);plot([0 1 1 0 0],[0 0 1 1 0]);disp('weights');
  Mux : Mux  Inputs=1
      mask Display: e = 0.06;c1 = [120 150 230]/255;c2 = ([120 150 230]+0)/383;c3 = ([120 150 230]+128)/383;patch([0 1 1 0],[0 0 1 1],c1);patch([0 1 1 1-e 1-e 0+e],[0 0 1 1-e 0+e 0+e],c2);patch([0 0 1 1-e 0+e 0+e],[0 1 1 1-e 1-e 0+e],c3);plot([0 1 1 0 0],[0 0 1 1 0]);disp('Mux');
  Subsystem : Subsystem
  "lz{2,1}" : Outport
      mask Display: e = 0.06;c1 = [120 230 180]/255;c2 = ([120 230 180]+0)/(256+128);c3 = ([120 230 180]+128)/(256+128);patch([0 1 1 0],[0 0 1 1],c1);patch([0 1 1 1-e 1-e 0+e],[0 0 1 1-e 0+e 0+e],c2);patch([0 0 1 1-e 0+e 0+e],[0 1 1 1-e 1-e 0+e],c3);plot([0 1 1 0 0],[0 0 1 1 0]);
  wires:
  Mux/1 -> "lz{2,1}"/1
  "IW{2,1}(1,:)'"/1 -> Subsystem/1(In1)
  "ad{2,1}"/1 -> Subsystem/2("ad{2,1}")
  Subsystem/1(Out1) -> Mux/1

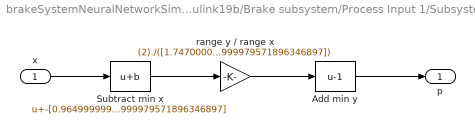
== system brakeSystemNeuralNetworkSimulink19b/Brake subsystem/Process Input 1/Subsystem ==
  x : Inport
  Add min y : Bias  Bias=-1
  Subtract min x : Bias  Bias=-[0.964999999999999968913755310496;3.31800000000000006039613253961;0.493999999999999994670929481799;0.476999999999999979571896346897]
  range y / range x : Gain  Gain=(2)./([1.74700000000000010835776720342;4.0929999999999999715782905696;1.08600000000000007638334409421;1.08099999999999996092014953319]-[0.964999999999999968913755310496;3.31800000000000006039613253961;0.493999999999999994670929481799;0.476999999999999979571896346897])
  p : Outport
  wires:
  range y / range x/1 -> Add min y/1
  Subtract min x/1 -> range y / range x/1
  x/1 -> Subtract min x/1
  Add min y/1 -> p/1

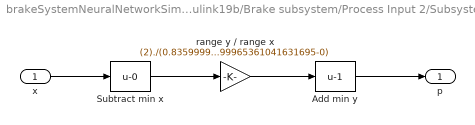
== system brakeSystemNeuralNetworkSimulink19b/Brake subsystem/Process Input 2/Subsystem ==
  x : Inport
  Add min y : Bias  Bias=-1
  Subtract min x : Bias  Bias=-0
  range y / range x : Gain  Gain=(2)./(0.835999999999999965361041631695-0)
  p : Outport
  wires:
  range y / range x/1 -> Add min y/1
  Subtract min x/1 -> range y / range x/1
  x/1 -> Subtract min x/1
  Add min y/1 -> p/1

== system brakeSystemNeuralNetworkSimulink19b/Brake subsystem/Process Output 1/Subsystem ==
  a : Inport
  Add min x : Bias
  Divide by range y : Gain  Gain=(0.835999999999999965361041631695-0)./(2)
  Subtract min y : Bias  Bias=1
  y : Outport
  wires:
  Divide by range y/1 -> Add min x/1
  Subtract min y/1 -> Divide by range y/1
  Add min x/1 -> y/1
  a/1 -> Subtract min y/1

== system brakeSystemNeuralNetworkSimulink19b/Brake subsystem/Layer 1/IW{1,1}/Subsystem ==
  In1 : Inport
  "pd{1,1}" : Inport  Port=2
  Dot Product : DotProduct  InputSameDT=on  OutDataTypeStr=Inherit: Inherit via internal rule
  Out1 : Outport
  wires:
  Dot Product/1 -> Out1/1
  In1/1 -> Dot Product/1
  "pd{1,1}"/1 -> Dot Product/2

== system brakeSystemNeuralNetworkSimulink19b/Brake subsystem/Layer 1/IW{1,1}/Subsystem1 ==
  In1 : Inport
  "pd{1,1}" : Inport  Port=2
  Dot Product : DotProduct  InputSameDT=on  OutDataTypeStr=Inherit: Inherit via internal rule
  Out1 : Outport
  wires:
  "pd{1,1}"/1 -> Dot Product/2
  In1/1 -> Dot Product/1
  Dot Product/1 -> Out1/1

== system brakeSystemNeuralNetworkSimulink19b/Brake subsystem/Layer 1/IW{1,1}/Subsystem2 ==
  In1 : Inport
  "pd{1,1}" : Inport  Port=2
  Dot Product : DotProduct  InputSameDT=on  OutDataTypeStr=Inherit: Inherit via internal rule
  Out1 : Outport
  wires:
  "pd{1,1}"/1 -> Dot Product/2
  In1/1 -> Dot Product/1
  Dot Product/1 -> Out1/1

== system brakeSystemNeuralNetworkSimulink19b/Brake subsystem/Layer 1/IW{1,1}/Subsystem3 ==
  In1 : Inport
  "pd{1,1}" : Inport  Port=2
  Dot Product : DotProduct  InputSameDT=on  OutDataTypeStr=Inherit: Inherit via internal rule
  Out1 : Outport
  wires:
  Dot Product/1 -> Out1/1
  In1/1 -> Dot Product/1
  "pd{1,1}"/1 -> Dot Product/2

== system brakeSystemNeuralNetworkSimulink19b/Brake subsystem/Layer 1/IW{1,1}/Subsystem4 ==
  In1 : Inport
  "pd{1,1}" : Inport  Port=2
  Dot Product : DotProduct  InputSameDT=on  OutDataTypeStr=Inherit: Inherit via internal rule
  Out1 : Outport
  wires:
  Dot Product/1 -> Out1/1
  In1/1 -> Dot Product/1
  "pd{1,1}"/1 -> Dot Product/2

== system brakeSystemNeuralNetworkSimulink19b/Brake subsystem/Layer 1/IW{1,1}/Subsystem5 ==
  In1 : Inport
  "pd{1,1}" : Inport  Port=2
  Dot Product : DotProduct  InputSameDT=on  OutDataTypeStr=Inherit: Inherit via internal rule
  Out1 : Outport
  wires:
  "pd{1,1}"/1 -> Dot Product/2
  Dot Product/1 -> Out1/1
  In1/1 -> Dot Product/1

== system brakeSystemNeuralNetworkSimulink19b/Brake subsystem/Layer 1/IW{1,2}/Subsystem ==
  In1 : Inport
  "pd{1,2}" : Inport  Port=2
  Dot Product : DotProduct  InputSameDT=on  OutDataTypeStr=Inherit: Inherit via internal rule
  Out1 : Outport
  wires:
  Dot Product/1 -> Out1/1
  In1/1 -> Dot Product/1
  "pd{1,2}"/1 -> Dot Product/2

== system brakeSystemNeuralNetworkSimulink19b/Brake subsystem/Layer 1/IW{1,2}/Subsystem1 ==
  In1 : Inport
  "pd{1,2}" : Inport  Port=2
  Dot Product : DotProduct  InputSameDT=on  OutDataTypeStr=Inherit: Inherit via internal rule
  Out1 : Outport
  wires:
  Dot Product/1 -> Out1/1
  In1/1 -> Dot Product/1
  "pd{1,2}"/1 -> Dot Product/2

== system brakeSystemNeuralNetworkSimulink19b/Brake subsystem/Layer 1/IW{1,2}/Subsystem2 ==
  In1 : Inport
  "pd{1,2}" : Inport  Port=2
  Dot Product : DotProduct  InputSameDT=on  OutDataTypeStr=Inherit: Inherit via internal rule
  Out1 : Outport
  wires:
  "pd{1,2}"/1 -> Dot Product/2
  Dot Product/1 -> Out1/1
  In1/1 -> Dot Product/1

== system brakeSystemNeuralNetworkSimulink19b/Brake subsystem/Layer 1/IW{1,2}/Subsystem3 ==
  In1 : Inport
  "pd{1,2}" : Inport  Port=2
  Dot Product : DotProduct  InputSameDT=on  OutDataTypeStr=Inherit: Inherit via internal rule
  Out1 : Outport
  wires:
  In1/1 -> Dot Product/1
  "pd{1,2}"/1 -> Dot Product/2
  Dot Product/1 -> Out1/1

== system brakeSystemNeuralNetworkSimulink19b/Brake subsystem/Layer 1/IW{1,2}/Subsystem4 ==
  In1 : Inport
  "pd{1,2}" : Inport  Port=2
  Dot Product : DotProduct  InputSameDT=on  OutDataTypeStr=Inherit: Inherit via internal rule
  Out1 : Outport
  wires:
  Dot Product/1 -> Out1/1
  "pd{1,2}"/1 -> Dot Product/2
  In1/1 -> Dot Product/1

== system brakeSystemNeuralNetworkSimulink19b/Brake subsystem/Layer 1/IW{1,2}/Subsystem5 ==
  In1 : Inport
  "pd{1,2}" : Inport  Port=2
  Dot Product : DotProduct  InputSameDT=on  OutDataTypeStr=Inherit: Inherit via internal rule
  Out1 : Outport
  wires:
  Dot Product/1 -> Out1/1
  "pd{1,2}"/1 -> Dot Product/2
  In1/1 -> Dot Product/1

== system brakeSystemNeuralNetworkSimulink19b/Brake subsystem/Layer 2/LW{2,1}/Subsystem ==
  In1 : Inport
  "ad{2,1}" : Inport  Port=2
  Dot Product : DotProduct  InputSameDT=on  OutDataTypeStr=Inherit: Inherit via internal rule
  Out1 : Outport
  wires:
  Dot Product/1 -> Out1/1
  In1/1 -> Dot Product/1
  "ad{2,1}"/1 -> Dot Product/2
